simulink model "TST_EngReq_TrqLimCalc"  (R2016b)
settings: Solver=FixedStepDiscrete  StartTime=0.0  StopTime=simTime  FixedStep=sampleTime  RelTol=1e-3
values from neighbouring files (symbols this model uses):
  testCase = 1    [initTST_EngReq_TrqLimCalc_001.m]
libraries: simulink x3, UnitTest_Lib x1
settings Model: Creator=zhengjinyan  LastModifiedBy=zhengjinyan
settings DebuggingCC: SignalRangeChecking=error

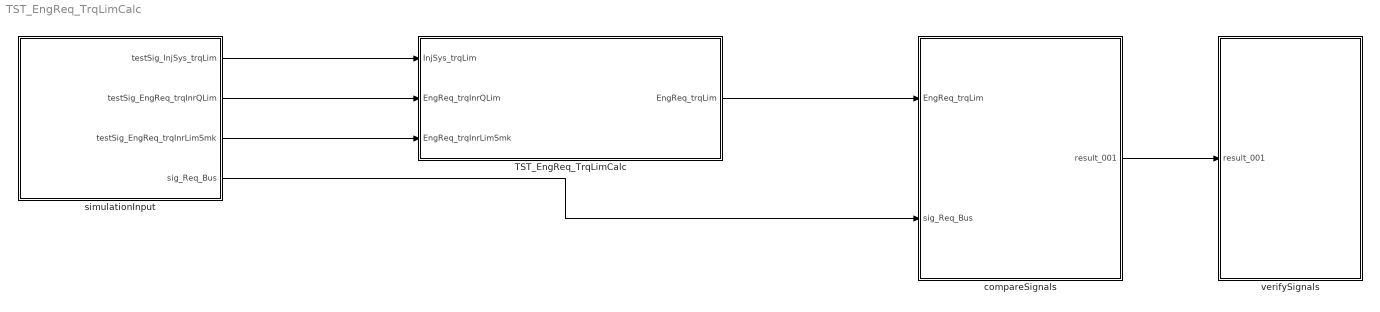
== system TST_EngReq_TrqLimCalc ==
  TST_EngReq_TrqLimCalc : Subsystem
  compareSignals : Subsystem
  simulationInput : Subsystem
  verifySignals : Subsystem
  wires:
  simulationInput/1(testSig_InjSys_trqLim) -> TST_EngReq_TrqLimCalc/1(InjSys_trqLim)
  simulationInput/2(testSig_EngReq_trqInrQLim) -> TST_EngReq_TrqLimCalc/2(EngReq_trqInrQLim)
  simulationInput/3(testSig_EngReq_trqInrLimSmk) -> TST_EngReq_TrqLimCalc/3(EngReq_trqInrLimSmk)
  TST_EngReq_TrqLimCalc/1(EngReq_trqLim) -> compareSignals/1(EngReq_trqLim)
  simulationInput/4(sig_Req_Bus) -> compareSignals/2(sig_Req_Bus)
  compareSignals/1(result_001) -> verifySignals/1(result_001)

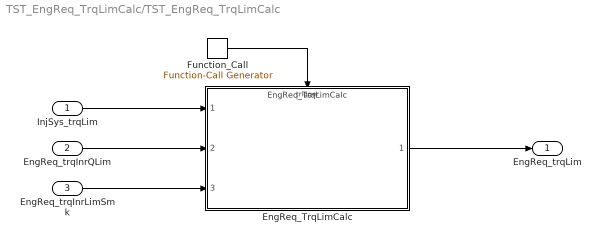
== system TST_EngReq_TrqLimCalc/TST_EngReq_TrqLimCalc ==
  InjSys_trqLim : Inport
  EngReq_trqInrQLim : Inport  Port=2
  EngReq_trqInrLimSmk : Inport  Port=3
  EngReq_TrqLimCalc : ModelReference  ModelNameDialog=EngReq_TrqLimCalc  SimulationMode=Normal  ModelReferenceVersion=1.11  TriggerPortName=function  TriggerPortTriggerType=function-call  TriggerPortStatesWhenEnabling=held
  Function_Call : simulink/Ports & Subsystems/Function-Call Generator  sample_time=sampleTime  numberOfIterations=1
  EngReq_trqLim : Outport
  wires:
  Function_Call/1 -> EngReq_TrqLimCalc/Trigger
  InjSys_trqLim/1 -> EngReq_TrqLimCalc/1
  EngReq_trqInrQLim/1 -> EngReq_TrqLimCalc/2
  EngReq_trqInrLimSmk/1 -> EngReq_TrqLimCalc/3
  EngReq_TrqLimCalc/1 -> EngReq_trqLim/1

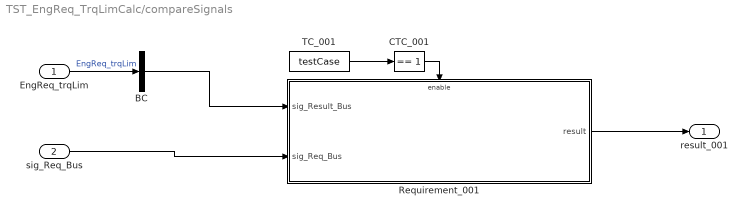
== system TST_EngReq_TrqLimCalc/compareSignals ==
  EngReq_trqLim : Inport
  sig_Req_Bus : Inport  Port=2
  BC : BusCreator  Inputs=1
  CTC_001 : simulink/Logic and Bit Operations/Compare To Constant  relop===  const=1  OutDataTypeStr=boolean
  Requirement_001 : Subsystem
  TC_001 : Constant  Value=testCase
  result_001 : Outport
  wires:
  EngReq_trqLim/1 -> BC/1  "EngReq_trqLim"
  TC_001/1 -> CTC_001/1
  CTC_001/1 -> Requirement_001/Enable
  sig_Req_Bus/1 -> Requirement_001/2(sig_Req_Bus)
  BC/1 -> Requirement_001/1(sig_Result_Bus)
  Requirement_001/1(result) -> result_001/1

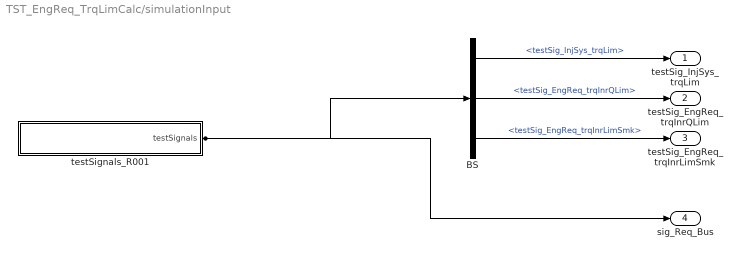
== system TST_EngReq_TrqLimCalc/simulationInput ==
  BS : BusSelector  OutputSignals=testSig_InjSys_trqLim,testSig_EngReq_trqInrQLim,testSig_EngReq_trqInrLimSmk
  testSignals_R001 : Subsystem
  testSig_InjSys_trqLim : Outport
  testSig_EngReq_trqInrQLim : Outport  Port=2
  testSig_EngReq_trqInrLimSmk : Outport  Port=3
  sig_Req_Bus : Outport  Port=4
  wires:
  BS/1 -> testSig_InjSys_trqLim/1  "<testSig_InjSys_trqLim>"
  BS/2 -> testSig_EngReq_trqInrQLim/1  "<testSig_EngReq_trqInrQLim>"
  BS/3 -> testSig_EngReq_trqInrLimSmk/1  "<testSig_EngReq_trqInrLimSmk>"
  testSignals_R001/1(testSignals) -> BS/1, sig_Req_Bus/1

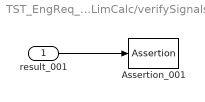
== system TST_EngReq_TrqLimCalc/verifySignals ==
  result_001 : Inport
  Assertion_001 : Assertion  Enabled=off
  wires:
  result_001/1 -> Assertion_001/1

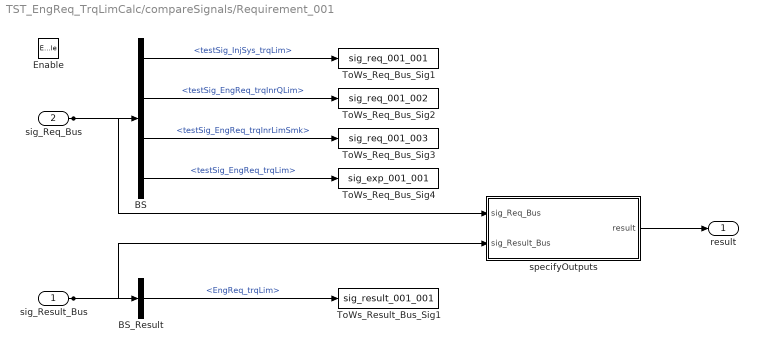
== system TST_EngReq_TrqLimCalc/compareSignals/Requirement_001 ==
  sig_Result_Bus : Inport
  sig_Req_Bus : Inport  Port=2
  Enable : EnablePort
  BS : BusSelector  OutputSignals=testSig_InjSys_trqLim,testSig_EngReq_trqInrQLim,testSig_EngReq_trqInrLimSmk,testSig_EngReq_trqLim
  BS_Result : BusSelector  OutputSignals=EngReq_trqLim
  ToWs_Req_Bus_Sig1 : ToWorkspace  VariableName=sig_req_001_001  SaveFormat=Structure With Time
  ToWs_Req_Bus_Sig2 : ToWorkspace  VariableName=sig_req_001_002  SaveFormat=Structure With Time
  ToWs_Req_Bus_Sig3 : ToWorkspace  VariableName=sig_req_001_003  SaveFormat=Structure With Time
  ToWs_Req_Bus_Sig4 : ToWorkspace  VariableName=sig_exp_001_001  SaveFormat=Structure With Time
  ToWs_Result_Bus_Sig1 : ToWorkspace  VariableName=sig_result_001_001  SaveFormat=Structure With Time
  specifyOutputs : Subsystem
  result : Outport
  wires:
  sig_Req_Bus/1 -> BS/1, specifyOutputs/1(sig_Req_Bus)
  BS/1 -> ToWs_Req_Bus_Sig1/1  "<testSig_InjSys_trqLim>"
  BS/2 -> ToWs_Req_Bus_Sig2/1  "<testSig_EngReq_trqInrQLim>"
  BS/3 -> ToWs_Req_Bus_Sig3/1  "<testSig_EngReq_trqInrLimSmk>"
  BS/4 -> ToWs_Req_Bus_Sig4/1  "<testSig_EngReq_trqLim>"
  sig_Result_Bus/1 -> BS_Result/1, specifyOutputs/2(sig_Result_Bus)
  BS_Result/1 -> ToWs_Result_Bus_Sig1/1  "<EngReq_trqLim>"
  specifyOutputs/1(result) -> result/1

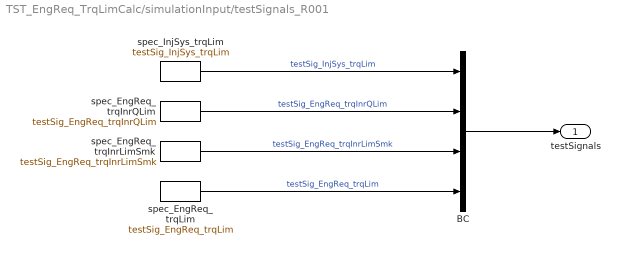
== system TST_EngReq_TrqLimCalc/simulationInput/testSignals_R001 ==
  BC : BusCreator  Inputs=4
  spec_EngReq_trqInrLimSmk : FromWorkspace  VariableName=testSig_EngReq_trqInrLimSmk  Interpolate=off  OutputAfterFinalValue=Holding final value
  spec_EngReq_trqInrQLim : FromWorkspace  VariableName=testSig_EngReq_trqInrQLim  Interpolate=off  OutputAfterFinalValue=Holding final value
  spec_EngReq_trqLim : FromWorkspace  VariableName=testSig_EngReq_trqLim  Interpolate=off  OutputAfterFinalValue=Holding final value
  spec_InjSys_trqLim : FromWorkspace  VariableName=testSig_InjSys_trqLim  Interpolate=off  OutputAfterFinalValue=Holding final value
  testSignals : Outport
  wires:
  BC/1 -> testSignals/1
  spec_InjSys_trqLim/1 -> BC/1  "testSig_InjSys_trqLim"
  spec_EngReq_trqInrQLim/1 -> BC/2  "testSig_EngReq_trqInrQLim"
  spec_EngReq_trqInrLimSmk/1 -> BC/3  "testSig_EngReq_trqInrLimSmk"
  spec_EngReq_trqLim/1 -> BC/4  "testSig_EngReq_trqLim"

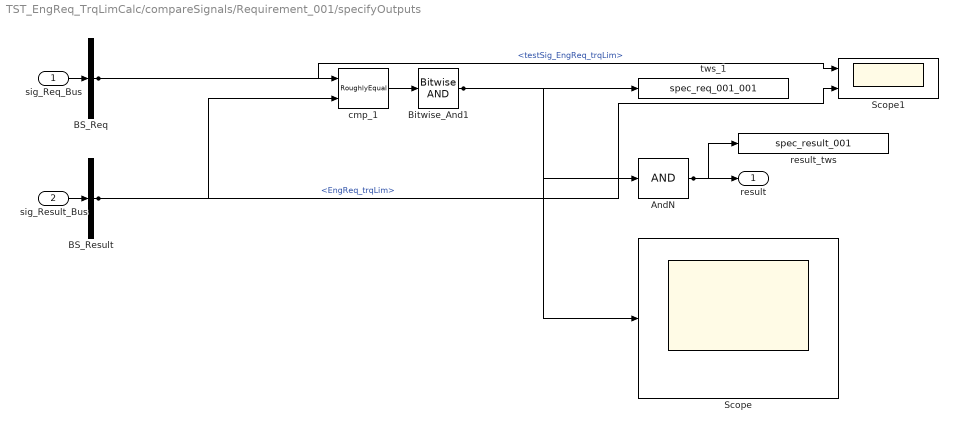
== system TST_EngReq_TrqLimCalc/compareSignals/Requirement_001/specifyOutputs ==
  sig_Req_Bus : Inport
  sig_Result_Bus : Inport  Port=2
  AndN : Logic  Inputs=1
  BS_Req : BusSelector  OutputSignals=testSig_EngReq_trqLim
  BS_Result : BusSelector  OutputSignals=EngReq_trqLim
  Bitwise_And1 : simulink/Logic and Bit Operations/Bitwise Operator  logicop=AND  UseBitMask=off  BitMask=bin2dec('11011001')  BitMaskRealWorld=Stored Integer
  Scope : Scope
  Scope1 : Scope  NumInputPorts=2
  cmp_1 : UnitTest_Lib/RoughlyEqual  slope=0.1
  result_tws : ToWorkspace  VariableName=spec_result_001
  tws_1 : ToWorkspace  VariableName=spec_req_001_001
  result : Outport
  wires:
  sig_Req_Bus/1 -> BS_Req/1
  sig_Result_Bus/1 -> BS_Result/1
  AndN/1 -> result/1, result_tws/1
  BS_Req/1 -> cmp_1/1, Scope1/1  "<testSig_EngReq_trqLim>"
  BS_Result/1 -> cmp_1/2, Scope1/2  "<EngReq_trqLim>"
  cmp_1/1 -> Bitwise_And1/1
  Bitwise_And1/1 -> tws_1/1, AndN/1, Scope/1
